simulink model "ebbers_moll_3"  (Simulink 7.4)
settings: Solver=ode23t  StartTime=0.0  StopTime=1e-6  MaxStep=1e-7  RelTol=1e-5
libraries: powerlib x71, simulink x1
settings Model: Creator=Dick Benson  LastModifiedBy=Dick
settings SolverCC: ZeroCrossControl=EnableAll
settings OptimizationCC: InlineInvariantSignals=on  InitFltsAndDblsToZero=on
settings DebuggingCC: AlgebraicLoopMsg=none  SaveWithParameterizedLinksMsg=none  SignalResolutionControl=TryResolveAllWithWarning  MultiTaskDSMMsg=warning  MultiTaskCondExecSysMsg=none  StrictBusMsg=None
settings RTWCC: IncludeERTFirstTime=on
settings GRTTargetCC: TargetFcnLib=ansi_tfl_tmw.mat

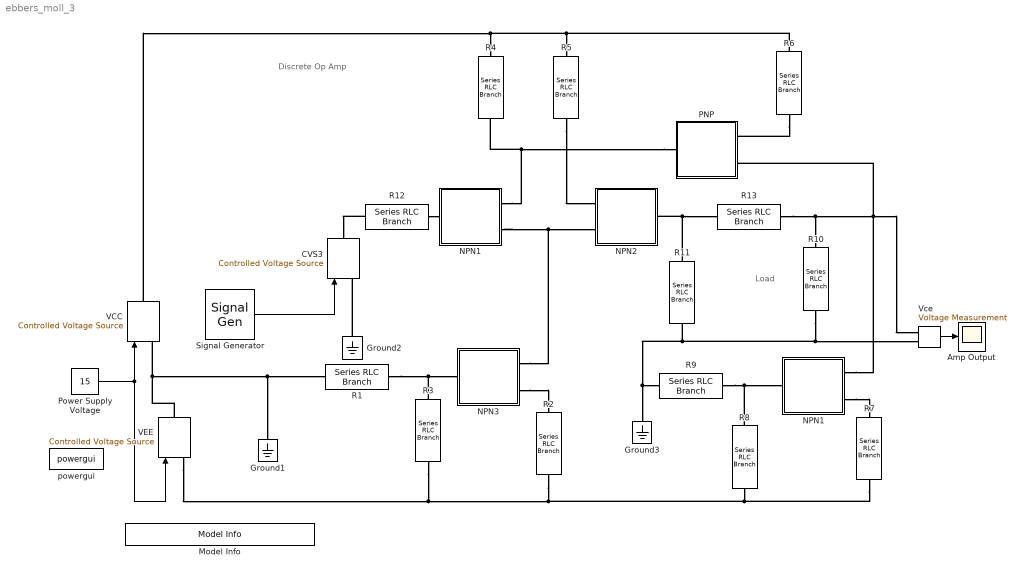
== system ebbers_moll_3 ==
  note: Discrete Op Amp
  note: Load
  " Power Supply Voltage" : Constant  Value=15  OutDataType=sfix(16)  OutScaling=2^0
  Amp Output : Scope
      settings: TimeRange=1e-006  YMin=-1.86228  YMax=1.74251  MaxDataPoints=50000
  CVS3 : powerlib/Electrical Sources/Controlled Voltage Source  DialogController=POWERSYS.PowerSysDialog  SystemSampleTime=-1  Initialize=on  Source_Type=AC  Amplitude=0  Phase=0  Frequency=0  Measurements=None
  Ground1 : powerlib/Elements/Ground  DialogController=POWERSYS.PowerSysDialog  PhysicalDomain=powersysdomain  SubClassName=unknown  LeftPortType=p1  RightPortType=p1  LConnTagsString=a
  Ground2 : powerlib/Elements/Ground  DialogController=POWERSYS.PowerSysDialog  PhysicalDomain=powersysdomain  SubClassName=unknown  LeftPortType=p1  RightPortType=p1  LConnTagsString=a
  Ground3 : powerlib/Elements/Ground  DialogController=POWERSYS.PowerSysDialog  PhysicalDomain=powersysdomain  SubClassName=unknown  LeftPortType=p1  RightPortType=p1  LConnTagsString=a
  Model Info : simulink/Model-Wide Utilities/Model Info  SystemSampleTime=-1  InitialBlockCM=None  BlockCM=None  Frame=on  DisplayStringWithTags=Copywrite 2005-2010 The MathWorks, Inc.  HorizontalTextAlignment=Center  LeftAlignmentValue=0.5  SourceBlockDiagram=ebbers_moll_3  TagMaxNumber=20
  NPN1 : Subsystem  mask{Beta=100, IEs=1e-10;, ICs=1e-10;, Ro=1e5, Cbc=5e-12, Cbe=50e-12, Rbb=100}
      mask init:
      | k = 1.38e-23;
      | q = 1.6e-19;
      | T = 290;
      | Vt = k*T/q;
  "NPN1 " : Subsystem  mask{Beta=40, IEs=1e-10;, ICs=1e-10;, Ro=1e5, Cbc=5e-12, Cbe=50e-12, Rbb=100}
      mask init:
      | k = 1.38e-23;
      | q = 1.6e-19;
      | T = 290;
      | Vt = k*T/q;
  NPN2 : Subsystem  mask{Beta=40, IEs=1e-10;, ICs=1e-10;, Ro=1e5, Cbc=5e-12, Cbe=50e-12, Rbb=100}
      mask init:
      | k = 1.38e-23;
      | q = 1.6e-19;
      | T = 290;
      | Vt = k*T/q;
  NPN3 : Subsystem  mask{Beta=100, IEs=1e-10;, ICs=1e-10;, Ro=1e5, Cbc=5e-12, Cbe=50e-12, Rbb=100}
      mask init:
      | k = 1.38e-23;
      | q = 1.6e-19;
      | T = 290;
      | Vt = k*T/q;
  PNP : Subsystem  mask{Beta=100, IEs=1e-8;, ICs=1e-8;, Ro=1e5, Cbc=5e-12, Cbe=50e-12, Rbb=100}
      mask init:
      | k = 1.38e-23;
      | q = 1.6e-19;
      | T = 290;
      | Vt = k*T/q;
  R{1,3,8..9} (4 alike) : powerlib/Elements/Series RLC Branch  DialogController=POWERSYS.PowerSysDialog  PhysicalDomain=powersysdomain  SubClassName=unknown  LeftPortType=p1  RightPortType=p1  LConnTagsString=__new0  RConnTagsString=__new0  BranchType=R  Resistance=1000  Inductance=1.0  SetiL0=off  InitialCurrent=0  Capacitance=1.0  Setx0=off  InitialVoltage=0  Measurements=None
  R10 : powerlib/Elements/Series RLC Branch  DialogController=POWERSYS.PowerSysDialog  PhysicalDomain=powersysdomain  SubClassName=unknown  LeftPortType=p1  RightPortType=p1  LConnTagsString=__new0  RConnTagsString=__new0  BranchType=R  Resistance=50  Inductance=1.0  SetiL0=off  InitialCurrent=0  Capacitance=1.0  Setx0=off  InitialVoltage=0  Measurements=None
  R11 : powerlib/Elements/Series RLC Branch  DialogController=POWERSYS.PowerSysDialog  PhysicalDomain=powersysdomain  SubClassName=unknown  LeftPortType=p1  RightPortType=p1  LConnTagsString=__new0  RConnTagsString=__new0  BranchType=R  Resistance=250  Inductance=1.0  SetiL0=off  InitialCurrent=0  Capacitance=1.0  Setx0=off  InitialVoltage=0  Measurements=None
  R12 : powerlib/Elements/Series RLC Branch  DialogController=POWERSYS.PowerSysDialog  PhysicalDomain=powersysdomain  SubClassName=unknown  LeftPortType=p1  RightPortType=p1  LConnTagsString=__new0  RConnTagsString=__new0  BranchType=R  Resistance=200  Inductance=1.0  SetiL0=off  InitialCurrent=0  Capacitance=1.0  Setx0=off  InitialVoltage=0  Measurements=None
  R13 : powerlib/Elements/Series RLC Branch  DialogController=POWERSYS.PowerSysDialog  PhysicalDomain=powersysdomain  SubClassName=unknown  LeftPortType=p1  RightPortType=p1  LConnTagsString=__new0  RConnTagsString=__new0  BranchType=R  Resistance=1200  Inductance=1.0  SetiL0=off  InitialCurrent=0  Capacitance=1.0  Setx0=off  InitialVoltage=0  Measurements=None
  R2 : powerlib/Elements/Series RLC Branch  DialogController=POWERSYS.PowerSysDialog  PhysicalDomain=powersysdomain  SubClassName=unknown  LeftPortType=p1  RightPortType=p1  LConnTagsString=__new0  RConnTagsString=__new0  BranchType=R  Resistance=330  Inductance=1.0  SetiL0=off  InitialCurrent=0  Capacitance=1.0  Setx0=off  InitialVoltage=0  Measurements=None
  R4 : powerlib/Elements/Series RLC Branch  DialogController=POWERSYS.PowerSysDialog  PhysicalDomain=powersysdomain  SubClassName=unknown  LeftPortType=p1  RightPortType=p1  LConnTagsString=__new0  RConnTagsString=__new0  BranchType=R  Resistance=200  Inductance=1.0  SetiL0=off  InitialCurrent=0  Capacitance=1.0  Setx0=off  InitialVoltage=0  Measurements=None
  R5 : powerlib/Elements/Series RLC Branch  DialogController=POWERSYS.PowerSysDialog  PhysicalDomain=powersysdomain  SubClassName=unknown  LeftPortType=p1  RightPortType=p1  LConnTagsString=__new0  RConnTagsString=__new0  BranchType=R  Resistance=200  Inductance=1.0  SetiL0=off  InitialCurrent=0  Capacitance=1.0  Setx0=off  InitialVoltage=0  Measurements=None
  R6 : powerlib/Elements/Series RLC Branch  DialogController=POWERSYS.PowerSysDialog  PhysicalDomain=powersysdomain  SubClassName=unknown  LeftPortType=p1  RightPortType=p1  LConnTagsString=__new0  RConnTagsString=__new0  BranchType=R  Resistance=10  Inductance=1.0  SetiL0=off  InitialCurrent=0  Capacitance=1.0  Setx0=off  InitialVoltage=0  Measurements=None
  R7 : powerlib/Elements/Series RLC Branch  DialogController=POWERSYS.PowerSysDialog  PhysicalDomain=powersysdomain  SubClassName=unknown  LeftPortType=p1  RightPortType=p1  LConnTagsString=__new0  RConnTagsString=__new0  BranchType=R  Resistance=50.35  Inductance=1.0  SetiL0=off  InitialCurrent=0  Capacitance=1.0  Setx0=off  InitialVoltage=0  Measurements=None
  Signal Generator : SignalGenerator  WaveForm=square  Amplitude=.2  Frequency=1e6
  VCC : powerlib/Electrical Sources/Controlled Voltage Source  DialogController=POWERSYS.PowerSysDialog  SystemSampleTime=-1  Initialize=on  Source_Type=DC  Amplitude=0  Phase=0  Frequency=0  Measurements=None
  VEE : powerlib/Electrical Sources/Controlled Voltage Source  DialogController=POWERSYS.PowerSysDialog  SystemSampleTime=-1  Initialize=on  Source_Type=DC  Amplitude=0  Phase=0  Frequency=0  Measurements=None
  "Vce " : powerlib/Measurements/Voltage Measurement  DialogController=POWERSYS.PowerSysDialog  SystemSampleTime=-1  PhasorSimulation=off  OutputType=Complex  PSBequivalent=0
  powergui : powerlib/powergui  SystemSampleTime=-1  SimulationMode=Continuous  SampleTime=0  frequency=60  SPID=off  DisableSnubberDevices=off  DisableRonSwitches=off  DisableVfSwitches=off  SwTol=0  Interpol=off  frequencyindice=0  echomessages=off  HookPort=off  DisplayEquations=off  FunctionMessages=off  EnableUseOfTLC=off  x0status=blocks  RestoreLinks=warning  Frange=[0:2:500]  Ylog=off  Xlog=on  ShowGrid=off  save=off  variable=ZData  ZoomFFT=on  StartTime=0.0  cycles=1  DisplayStyle=1  fundamental=60  FreqAxis=off  MaxFrequency=1000  frequencyindicesteady=1  RmsSteady=1  display=off  Ts=0  methode=off
  wires:
  "Vce "/1 -> Amp Output/1
  " Power Supply Voltage"/1 -> VCC/1, VEE/1
  Signal Generator/1 -> CVS3/1
  connections:
  VEE/LConn1 -- R7/RConn1 -- R8/RConn1 -- R2/RConn1 -- R3/RConn1
  NPN3/RConn2 -- R2/LConn1
  R3/LConn1 -- NPN3/LConn1 -- R1/RConn1
  "NPN1 "/RConn2 -- NPN2/RConn2 -- NPN3/RConn1
  PNP/LConn1 -- "NPN1 "/RConn1 -- R4/RConn1
  R5/RConn1 -- NPN2/RConn1
  R6/LConn1 -- VCC/RConn1 -- R4/LConn1 -- R5/LConn1
  VEE/RConn1 -- VCC/LConn1 -- R1/LConn1 -- Ground1/LConn1
  Ground2/LConn1 -- CVS3/LConn1
  R6/RConn1 -- PNP/RConn1
  R11/RConn1 -- R10/RConn1 -- "Vce "/LConn2 -- Ground3/LConn1 -- R9/LConn1
  NPN1/RConn2 -- R7/LConn1
  R8/LConn1 -- NPN1/LConn1 -- R9/RConn1
  R11/LConn1 -- NPN2/LConn1 -- R13/LConn1
  R12/LConn1 -- "NPN1 "/LConn1
  R12/RConn1 -- CVS3/RConn1
  R10/LConn1 -- R13/RConn1 -- PNP/RConn2 -- NPN1/RConn1 -- "Vce "/LConn1

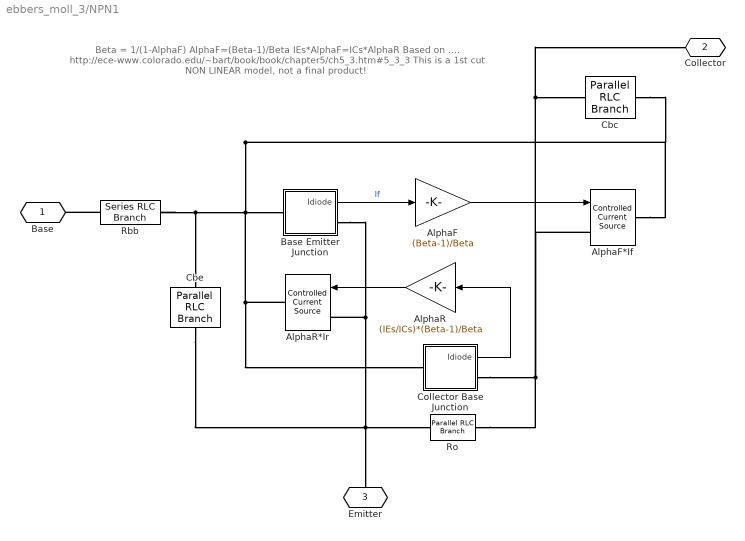
== system ebbers_moll_3/NPN1 ==
  note: Beta = 1/(1-AlphaF)
      | AlphaF=(Beta-1)/Beta
      | IEs*AlphaF=ICs*AlphaR
      |
      | Based on ....
      | http://ece-www.colorado.edu/~bart/book/book/chapter5/ch5_3.htm#5_3_3
      |
      | This is a 1st cut NON LINEAR model, not a final product!
  AlphaF : Gain  Gain=(Beta-1)/Beta  ParameterDataType=sfix(16)  ParameterScaling=2^0  OutDataType=sfix(16)  OutScaling=2^0
  AlphaF*If : powerlib/Electrical Sources/Controlled Current Source  Description=source block  DialogController=POWERSYS.PowerSysDialog  SystemSampleTime=-1  Initialize=off  Source_Type=AC  Amplitude=-0.025  Phase=0  Frequency=0  Measurements=None
      settings: AttributesFormatString=\n
  AlphaR : Gain  Gain=(IEs/ICs)*(Beta-1)/Beta  ParameterDataType=sfix(16)  ParameterScaling=2^0  OutDataType=sfix(16)  OutScaling=2^0
  AlphaR*Ir : powerlib/Electrical Sources/Controlled Current Source  Description=source block  DialogController=POWERSYS.PowerSysDialog  SystemSampleTime=-1  Initialize=off  Source_Type=AC  Amplitude=-0.025  Phase=0  Frequency=0  Measurements=None
      settings: AttributesFormatString=\n
  Base Emitter Junction : Subsystem  AncestorBlock=simcircuits_library_1/diode  mask{Is=IEs}
      mask prompts: Is "Saturation Current"
      mask Display: plot(-140,-140,150,140,2*[30,30,59,30,30,0]-75,(2*[71,50,72,92,71,71]-92),2*[59,59]-75,(2*[50,93]-92),[116,59]-16,(2*[71,71]-90));
  Cbc : powerlib/Elements/Parallel RLC Branch  DialogController=POWERSYS.PowerSysDialog  PhysicalDomain=powersysdomain  SubClassName=unknown  LeftPortType=p1  RightPortType=p1  LConnTagsString=a  RConnTagsString=__new0  BranchType=C  Resistance=1.0  Inductance=1.0  SetiL0=off  InitialCurrent=0  Capacitance=Cbc  Setx0=off  InitialVoltage=0  Measurements=None
  Cbe : powerlib/Elements/Parallel RLC Branch  DialogController=POWERSYS.PowerSysDialog  PhysicalDomain=powersysdomain  SubClassName=unknown  LeftPortType=p1  RightPortType=p1  LConnTagsString=a  RConnTagsString=__new0  BranchType=C  Resistance=1.0  Inductance=1.0  SetiL0=off  InitialCurrent=0  Capacitance=Cbe  Setx0=off  InitialVoltage=0  Measurements=None
  Collector Base Junction : Subsystem  AncestorBlock=simcircuits_library_1/diode  mask{Is=ICs}
      mask prompts: Is "Saturation Current"
      mask Display: plot(-140,-140,150,140,2*[30,30,59,30,30,0]-75,(2*[71,50,72,92,71,71]-92),2*[59,59]-75,(2*[50,93]-92),[116,59]-16,(2*[71,71]-90));
  Rbb : powerlib/Elements/Series RLC Branch  DialogController=POWERSYS.PowerSysDialog  PhysicalDomain=powersysdomain  SubClassName=unknown  LeftPortType=p1  RightPortType=p1  LConnTagsString=__new0  RConnTagsString=__new0  BranchType=R  Resistance=Rbb  Inductance=1.0  SetiL0=off  InitialCurrent=0  Capacitance=1.0  Setx0=off  InitialVoltage=0  Measurements=None
  Ro : powerlib/Elements/Parallel RLC Branch  DialogController=POWERSYS.PowerSysDialog  PhysicalDomain=powersysdomain  SubClassName=unknown  LeftPortType=p1  RightPortType=p1  LConnTagsString=a  RConnTagsString=__new0  BranchType=R  Resistance=Ro  Inductance=1.0  SetiL0=off  InitialCurrent=0  Capacitance=1.0  Setx0=off  InitialVoltage=0  Measurements=None
  Base : PMIOPort  Port=1  Side=Left
  Collector : PMIOPort  Port=2  Side=Right
  Emitter : PMIOPort  Port=3  Side=Right
  wires:
  Base Emitter Junction/1(Idiode) -> AlphaF/1  "If"
  AlphaF/1 -> AlphaF*If/1
  Collector Base Junction/1(Idiode) -> AlphaR/1
  AlphaR/1 -> AlphaR*Ir/1
  connections:
  Rbb/RConn1 -- Cbe/LConn1 -- Base Emitter Junction/LConn1 -- AlphaF*If/RConn1 -- Cbc/RConn1 -- AlphaR*Ir/RConn1 -- Collector Base Junction/LConn1
  AlphaR*Ir/LConn1 -- Emitter/RConn1 -- Cbe/RConn1 -- Ro/LConn1 -- Base Emitter Junction/RConn1
  AlphaF*If/LConn1 -- Collector/RConn1 -- Cbc/LConn1 -- Collector Base Junction/RConn1 -- Ro/RConn1
  Rbb/LConn1 -- Base/RConn1

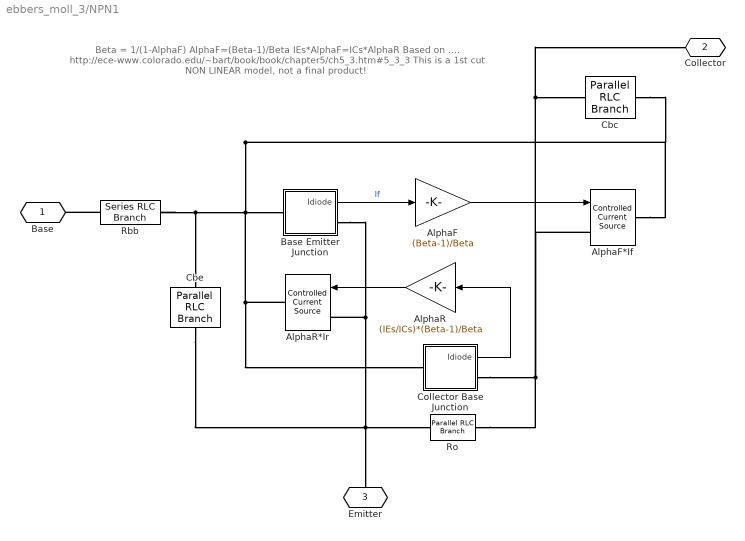
== system ebbers_moll_3/NPN1  ==
  note: Beta = 1/(1-AlphaF)
      | AlphaF=(Beta-1)/Beta
      | IEs*AlphaF=ICs*AlphaR
      |
      | Based on ....
      | http://ece-www.colorado.edu/~bart/book/book/chapter5/ch5_3.htm#5_3_3
      |
      | This is a 1st cut NON LINEAR model, not a final product!
  AlphaF : Gain  Gain=(Beta-1)/Beta  ParameterDataType=sfix(16)  ParameterScaling=2^0  OutDataType=sfix(16)  OutScaling=2^0
  AlphaF*If : powerlib/Electrical Sources/Controlled Current Source  Description=source block  DialogController=POWERSYS.PowerSysDialog  SystemSampleTime=-1  Initialize=off  Source_Type=AC  Amplitude=-0.025  Phase=0  Frequency=0  Measurements=None
      settings: AttributesFormatString=\n
  AlphaR : Gain  Gain=(IEs/ICs)*(Beta-1)/Beta  ParameterDataType=sfix(16)  ParameterScaling=2^0  OutDataType=sfix(16)  OutScaling=2^0
  AlphaR*Ir : powerlib/Electrical Sources/Controlled Current Source  Description=source block  DialogController=POWERSYS.PowerSysDialog  SystemSampleTime=-1  Initialize=off  Source_Type=AC  Amplitude=-0.025  Phase=0  Frequency=0  Measurements=None
      settings: AttributesFormatString=\n
  Base Emitter Junction : Subsystem  AncestorBlock=simcircuits_library_1/diode  mask{Is=IEs}
      mask prompts: Is "Saturation Current"
      mask Display: plot(-140,-140,150,140,2*[30,30,59,30,30,0]-75,(2*[71,50,72,92,71,71]-92),2*[59,59]-75,(2*[50,93]-92),[116,59]-16,(2*[71,71]-90));
  Cbc : powerlib/Elements/Parallel RLC Branch  DialogController=POWERSYS.PowerSysDialog  PhysicalDomain=powersysdomain  SubClassName=unknown  LeftPortType=p1  RightPortType=p1  LConnTagsString=a  RConnTagsString=__new0  BranchType=C  Resistance=1.0  Inductance=1.0  SetiL0=off  InitialCurrent=0  Capacitance=Cbc  Setx0=off  InitialVoltage=0  Measurements=None
  Cbe : powerlib/Elements/Parallel RLC Branch  DialogController=POWERSYS.PowerSysDialog  PhysicalDomain=powersysdomain  SubClassName=unknown  LeftPortType=p1  RightPortType=p1  LConnTagsString=a  RConnTagsString=__new0  BranchType=C  Resistance=1.0  Inductance=1.0  SetiL0=off  InitialCurrent=0  Capacitance=Cbe  Setx0=off  InitialVoltage=0  Measurements=None
  Collector Base Junction : Subsystem  AncestorBlock=simcircuits_library_1/diode  mask{Is=ICs}
      mask prompts: Is "Saturation Current"
      mask Display: plot(-140,-140,150,140,2*[30,30,59,30,30,0]-75,(2*[71,50,72,92,71,71]-92),2*[59,59]-75,(2*[50,93]-92),[116,59]-16,(2*[71,71]-90));
  Rbb : powerlib/Elements/Series RLC Branch  DialogController=POWERSYS.PowerSysDialog  PhysicalDomain=powersysdomain  SubClassName=unknown  LeftPortType=p1  RightPortType=p1  LConnTagsString=__new0  RConnTagsString=__new0  BranchType=R  Resistance=Rbb  Inductance=1.0  SetiL0=off  InitialCurrent=0  Capacitance=1.0  Setx0=off  InitialVoltage=0  Measurements=None
  Ro : powerlib/Elements/Parallel RLC Branch  DialogController=POWERSYS.PowerSysDialog  PhysicalDomain=powersysdomain  SubClassName=unknown  LeftPortType=p1  RightPortType=p1  LConnTagsString=a  RConnTagsString=__new0  BranchType=R  Resistance=Ro  Inductance=1.0  SetiL0=off  InitialCurrent=0  Capacitance=1.0  Setx0=off  InitialVoltage=0  Measurements=None
  Base : PMIOPort  Port=1  Side=Left
  Collector : PMIOPort  Port=2  Side=Right
  Emitter : PMIOPort  Port=3  Side=Right
  wires:
  Base Emitter Junction/1(Idiode) -> AlphaF/1  "If"
  AlphaF/1 -> AlphaF*If/1
  Collector Base Junction/1(Idiode) -> AlphaR/1
  AlphaR/1 -> AlphaR*Ir/1
  connections:
  Rbb/RConn1 -- Cbe/LConn1 -- Base Emitter Junction/LConn1 -- AlphaF*If/RConn1 -- Cbc/RConn1 -- AlphaR*Ir/RConn1 -- Collector Base Junction/LConn1
  AlphaR*Ir/LConn1 -- Emitter/RConn1 -- Cbe/RConn1 -- Ro/LConn1 -- Base Emitter Junction/RConn1
  AlphaF*If/LConn1 -- Collector/RConn1 -- Cbc/LConn1 -- Collector Base Junction/RConn1 -- Ro/RConn1
  Rbb/LConn1 -- Base/RConn1

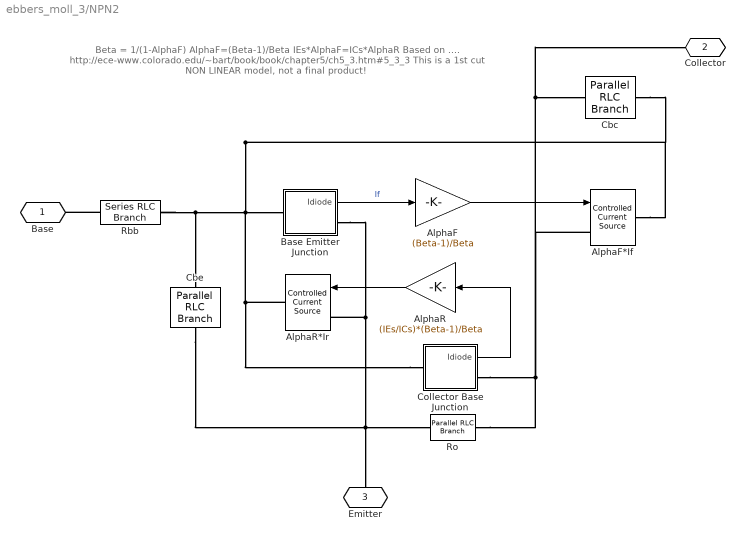
== system ebbers_moll_3/NPN2 ==
  note: Beta = 1/(1-AlphaF)
      | AlphaF=(Beta-1)/Beta
      | IEs*AlphaF=ICs*AlphaR
      |
      | Based on ....
      | http://ece-www.colorado.edu/~bart/book/book/chapter5/ch5_3.htm#5_3_3
      |
      | This is a 1st cut NON LINEAR model, not a final product!
  AlphaF : Gain  Gain=(Beta-1)/Beta  ParameterDataType=sfix(16)  ParameterScaling=2^0  OutDataType=sfix(16)  OutScaling=2^0
  AlphaF*If : powerlib/Electrical Sources/Controlled Current Source  Description=source block  DialogController=POWERSYS.PowerSysDialog  SystemSampleTime=-1  Initialize=off  Source_Type=AC  Amplitude=-0.025  Phase=0  Frequency=0  Measurements=None
      settings: AttributesFormatString=\n
  AlphaR : Gain  Gain=(IEs/ICs)*(Beta-1)/Beta  ParameterDataType=sfix(16)  ParameterScaling=2^0  OutDataType=sfix(16)  OutScaling=2^0
  AlphaR*Ir : powerlib/Electrical Sources/Controlled Current Source  Description=source block  DialogController=POWERSYS.PowerSysDialog  SystemSampleTime=-1  Initialize=off  Source_Type=AC  Amplitude=-0.025  Phase=0  Frequency=0  Measurements=None
      settings: AttributesFormatString=\n
  Base Emitter Junction : Subsystem  AncestorBlock=simcircuits_library_1/diode  mask{Is=IEs}
      mask prompts: Is "Saturation Current"
      mask Display: plot(-140,-140,150,140,2*[30,30,59,30,30,0]-75,(2*[71,50,72,92,71,71]-92),2*[59,59]-75,(2*[50,93]-92),[116,59]-16,(2*[71,71]-90));
  Cbc : powerlib/Elements/Parallel RLC Branch  DialogController=POWERSYS.PowerSysDialog  PhysicalDomain=powersysdomain  SubClassName=unknown  LeftPortType=p1  RightPortType=p1  LConnTagsString=a  RConnTagsString=__new0  BranchType=C  Resistance=1.0  Inductance=1.0  SetiL0=off  InitialCurrent=0  Capacitance=Cbc  Setx0=off  InitialVoltage=0  Measurements=None
  Cbe : powerlib/Elements/Parallel RLC Branch  DialogController=POWERSYS.PowerSysDialog  PhysicalDomain=powersysdomain  SubClassName=unknown  LeftPortType=p1  RightPortType=p1  LConnTagsString=a  RConnTagsString=__new0  BranchType=C  Resistance=1.0  Inductance=1.0  SetiL0=off  InitialCurrent=0  Capacitance=Cbe  Setx0=off  InitialVoltage=0  Measurements=None
  Collector Base Junction : Subsystem  AncestorBlock=simcircuits_library_1/diode  mask{Is=ICs}
      mask prompts: Is "Saturation Current"
      mask Display: plot(-140,-140,150,140,2*[30,30,59,30,30,0]-75,(2*[71,50,72,92,71,71]-92),2*[59,59]-75,(2*[50,93]-92),[116,59]-16,(2*[71,71]-90));
  Rbb : powerlib/Elements/Series RLC Branch  DialogController=POWERSYS.PowerSysDialog  PhysicalDomain=powersysdomain  SubClassName=unknown  LeftPortType=p1  RightPortType=p1  LConnTagsString=__new0  RConnTagsString=__new0  BranchType=R  Resistance=Rbb  Inductance=1.0  SetiL0=off  InitialCurrent=0  Capacitance=1.0  Setx0=off  InitialVoltage=0  Measurements=None
  Ro : powerlib/Elements/Parallel RLC Branch  DialogController=POWERSYS.PowerSysDialog  PhysicalDomain=powersysdomain  SubClassName=unknown  LeftPortType=p1  RightPortType=p1  LConnTagsString=a  RConnTagsString=__new0  BranchType=R  Resistance=Ro  Inductance=1.0  SetiL0=off  InitialCurrent=0  Capacitance=1.0  Setx0=off  InitialVoltage=0  Measurements=None
  Base : PMIOPort  Port=1  Side=Left
  Collector : PMIOPort  Port=2  Side=Right
  Emitter : PMIOPort  Port=3  Side=Right
  wires:
  AlphaR/1 -> AlphaR*Ir/1
  Collector Base Junction/1(Idiode) -> AlphaR/1
  AlphaF/1 -> AlphaF*If/1
  Base Emitter Junction/1(Idiode) -> AlphaF/1  "If"
  connections:
  Rbb/LConn1 -- Base/RConn1
  Ro/RConn1 -- Collector Base Junction/RConn1 -- Cbc/LConn1 -- Collector/RConn1 -- AlphaF*If/LConn1
  Base Emitter Junction/RConn1 -- Ro/LConn1 -- Cbe/RConn1 -- Emitter/RConn1 -- AlphaR*Ir/LConn1
  Collector Base Junction/LConn1 -- AlphaR*Ir/RConn1 -- Cbc/RConn1 -- AlphaF*If/RConn1 -- Base Emitter Junction/LConn1 -- Cbe/LConn1 -- Rbb/RConn1

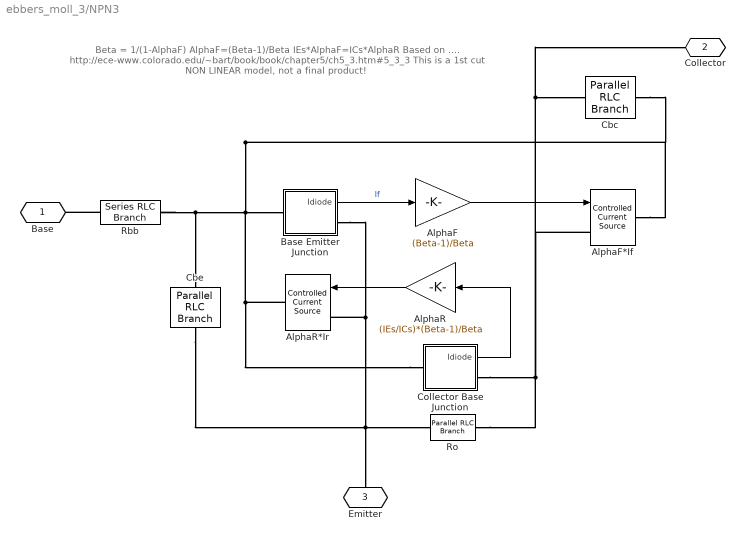
== system ebbers_moll_3/NPN3 ==
  note: Beta = 1/(1-AlphaF)
      | AlphaF=(Beta-1)/Beta
      | IEs*AlphaF=ICs*AlphaR
      |
      | Based on ....
      | http://ece-www.colorado.edu/~bart/book/book/chapter5/ch5_3.htm#5_3_3
      |
      | This is a 1st cut NON LINEAR model, not a final product!
  AlphaF : Gain  Gain=(Beta-1)/Beta  ParameterDataType=sfix(16)  ParameterScaling=2^0  OutDataType=sfix(16)  OutScaling=2^0
  AlphaF*If : powerlib/Electrical Sources/Controlled Current Source  Description=source block  DialogController=POWERSYS.PowerSysDialog  SystemSampleTime=-1  Initialize=off  Source_Type=AC  Amplitude=-0.025  Phase=0  Frequency=0  Measurements=None
      settings: AttributesFormatString=\n
  AlphaR : Gain  Gain=(IEs/ICs)*(Beta-1)/Beta  ParameterDataType=sfix(16)  ParameterScaling=2^0  OutDataType=sfix(16)  OutScaling=2^0
  AlphaR*Ir : powerlib/Electrical Sources/Controlled Current Source  Description=source block  DialogController=POWERSYS.PowerSysDialog  SystemSampleTime=-1  Initialize=off  Source_Type=AC  Amplitude=-0.025  Phase=0  Frequency=0  Measurements=None
      settings: AttributesFormatString=\n
  Base Emitter Junction : Subsystem  AncestorBlock=simcircuits_library_1/diode  mask{Is=IEs}
      mask prompts: Is "Saturation Current"
      mask Display: plot(-140,-140,150,140,2*[30,30,59,30,30,0]-75,(2*[71,50,72,92,71,71]-92),2*[59,59]-75,(2*[50,93]-92),[116,59]-16,(2*[71,71]-90));
  Cbc : powerlib/Elements/Parallel RLC Branch  DialogController=POWERSYS.PowerSysDialog  PhysicalDomain=powersysdomain  SubClassName=unknown  LeftPortType=p1  RightPortType=p1  LConnTagsString=a  RConnTagsString=__new0  BranchType=C  Resistance=1.0  Inductance=1.0  SetiL0=off  InitialCurrent=0  Capacitance=Cbc  Setx0=off  InitialVoltage=0  Measurements=None
  Cbe : powerlib/Elements/Parallel RLC Branch  DialogController=POWERSYS.PowerSysDialog  PhysicalDomain=powersysdomain  SubClassName=unknown  LeftPortType=p1  RightPortType=p1  LConnTagsString=a  RConnTagsString=__new0  BranchType=C  Resistance=1.0  Inductance=1.0  SetiL0=off  InitialCurrent=0  Capacitance=Cbe  Setx0=off  InitialVoltage=0  Measurements=None
  Collector Base Junction : Subsystem  AncestorBlock=simcircuits_library_1/diode  mask{Is=ICs}
      mask prompts: Is "Saturation Current"
      mask Display: plot(-140,-140,150,140,2*[30,30,59,30,30,0]-75,(2*[71,50,72,92,71,71]-92),2*[59,59]-75,(2*[50,93]-92),[116,59]-16,(2*[71,71]-90));
  Rbb : powerlib/Elements/Series RLC Branch  DialogController=POWERSYS.PowerSysDialog  PhysicalDomain=powersysdomain  SubClassName=unknown  LeftPortType=p1  RightPortType=p1  LConnTagsString=__new0  RConnTagsString=__new0  BranchType=R  Resistance=Rbb  Inductance=1.0  SetiL0=off  InitialCurrent=0  Capacitance=1.0  Setx0=off  InitialVoltage=0  Measurements=None
  Ro : powerlib/Elements/Parallel RLC Branch  DialogController=POWERSYS.PowerSysDialog  PhysicalDomain=powersysdomain  SubClassName=unknown  LeftPortType=p1  RightPortType=p1  LConnTagsString=a  RConnTagsString=__new0  BranchType=R  Resistance=Ro  Inductance=1.0  SetiL0=off  InitialCurrent=0  Capacitance=1.0  Setx0=off  InitialVoltage=0  Measurements=None
  Base : PMIOPort  Port=1  Side=Left
  Collector : PMIOPort  Port=2  Side=Right
  Emitter : PMIOPort  Port=3  Side=Right
  wires:
  AlphaR/1 -> AlphaR*Ir/1
  Collector Base Junction/1(Idiode) -> AlphaR/1
  AlphaF/1 -> AlphaF*If/1
  Base Emitter Junction/1(Idiode) -> AlphaF/1  "If"
  connections:
  Rbb/LConn1 -- Base/RConn1
  Ro/RConn1 -- Collector Base Junction/RConn1 -- Cbc/LConn1 -- Collector/RConn1 -- AlphaF*If/LConn1
  Base Emitter Junction/RConn1 -- Ro/LConn1 -- Cbe/RConn1 -- Emitter/RConn1 -- AlphaR*Ir/LConn1
  Collector Base Junction/LConn1 -- AlphaR*Ir/RConn1 -- Cbc/RConn1 -- AlphaF*If/RConn1 -- Base Emitter Junction/LConn1 -- Cbe/LConn1 -- Rbb/RConn1

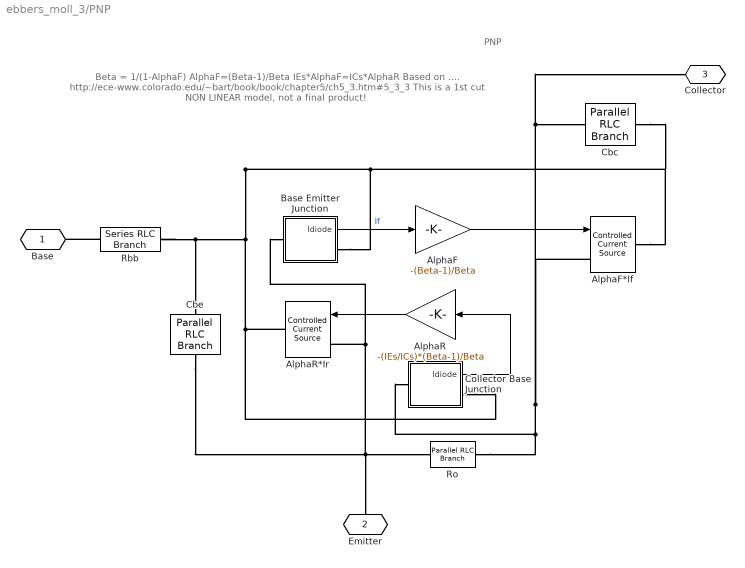
== system ebbers_moll_3/PNP ==
  note: Beta = 1/(1-AlphaF)
      | AlphaF=(Beta-1)/Beta
      | IEs*AlphaF=ICs*AlphaR
      |
      | Based on ....
      | http://ece-www.colorado.edu/~bart/book/book/chapter5/ch5_3.htm#5_3_3
      |
      | This is a 1st cut NON LINEAR model, not a final product!
  note: PNP
  AlphaF : Gain  Gain=-(Beta-1)/Beta  ParameterDataType=sfix(16)  ParameterScaling=2^0  OutDataType=sfix(16)  OutScaling=2^0
  AlphaF*If : powerlib/Electrical Sources/Controlled Current Source  Description=source block  DialogController=POWERSYS.PowerSysDialog  SystemSampleTime=-1  Initialize=off  Source_Type=AC  Amplitude=-0.025  Phase=0  Frequency=0  Measurements=None
      settings: AttributesFormatString=\n
  AlphaR : Gain  Gain=-(IEs/ICs)*(Beta-1)/Beta  ParameterDataType=sfix(16)  ParameterScaling=2^0  OutDataType=sfix(16)  OutScaling=2^0
  AlphaR*Ir : powerlib/Electrical Sources/Controlled Current Source  Description=source block  DialogController=POWERSYS.PowerSysDialog  SystemSampleTime=-1  Initialize=off  Source_Type=AC  Amplitude=-0.025  Phase=0  Frequency=0  Measurements=None
      settings: AttributesFormatString=\n
  Base Emitter Junction : Subsystem  AncestorBlock=simcircuits_library_1/diode  mask{Is=IEs}
      mask prompts: Is "Saturation Current"
      mask Display: plot(-140,-140,150,140,2*[30,30,59,30,30,0]-75,(2*[71,50,72,92,71,71]-92),2*[59,59]-75,(2*[50,93]-92),[116,59]-16,(2*[71,71]-90));
  Cbc : powerlib/Elements/Parallel RLC Branch  DialogController=POWERSYS.PowerSysDialog  PhysicalDomain=powersysdomain  SubClassName=unknown  LeftPortType=p1  RightPortType=p1  LConnTagsString=a  RConnTagsString=__new0  BranchType=C  Resistance=1.0  Inductance=1.0  SetiL0=off  InitialCurrent=0  Capacitance=Cbc  Setx0=off  InitialVoltage=0  Measurements=None
  Cbe : powerlib/Elements/Parallel RLC Branch  DialogController=POWERSYS.PowerSysDialog  PhysicalDomain=powersysdomain  SubClassName=unknown  LeftPortType=p1  RightPortType=p1  LConnTagsString=a  RConnTagsString=__new0  BranchType=C  Resistance=1.0  Inductance=1.0  SetiL0=off  InitialCurrent=0  Capacitance=Cbe  Setx0=off  InitialVoltage=0  Measurements=None
  Collector Base Junction : Subsystem  AncestorBlock=simcircuits_library_1/diode  mask{Is=ICs}
      mask prompts: Is "Saturation Current"
      mask Display: plot(-140,-140,150,140,2*[30,30,59,30,30,0]-75,(2*[71,50,72,92,71,71]-92),2*[59,59]-75,(2*[50,93]-92),[116,59]-16,(2*[71,71]-90));
  Rbb : powerlib/Elements/Series RLC Branch  DialogController=POWERSYS.PowerSysDialog  PhysicalDomain=powersysdomain  SubClassName=unknown  LeftPortType=p1  RightPortType=p1  LConnTagsString=__new0  RConnTagsString=__new0  BranchType=R  Resistance=Rbb  Inductance=1.0  SetiL0=off  InitialCurrent=0  Capacitance=1.0  Setx0=off  InitialVoltage=0  Measurements=None
  Ro : powerlib/Elements/Parallel RLC Branch  DialogController=POWERSYS.PowerSysDialog  PhysicalDomain=powersysdomain  SubClassName=unknown  LeftPortType=p1  RightPortType=p1  LConnTagsString=a  RConnTagsString=__new0  BranchType=R  Resistance=Ro  Inductance=1.0  SetiL0=off  InitialCurrent=0  Capacitance=1.0  Setx0=off  InitialVoltage=0  Measurements=None
  Base : PMIOPort  Port=1  Side=Left
  Emitter : PMIOPort  Port=2  Side=Right
  Collector : PMIOPort  Port=3  Side=Right
  wires:
  Base Emitter Junction/1(Idiode) -> AlphaF/1  "If"
  AlphaF/1 -> AlphaF*If/1
  Collector Base Junction/1(Idiode) -> AlphaR/1
  AlphaR/1 -> AlphaR*Ir/1
  connections:
  Collector Base Junction/RConn1 -- AlphaR*Ir/RConn1 -- Rbb/RConn1 -- Cbe/LConn1 -- AlphaF*If/RConn1 -- Cbc/RConn1 -- Base Emitter Junction/RConn1
  Emitter/RConn1 -- Cbe/RConn1 -- Ro/LConn1 -- AlphaR*Ir/LConn1 -- Base Emitter Junction/LConn1
  Ro/RConn1 -- AlphaF*If/LConn1 -- Collector/RConn1 -- Cbc/LConn1 -- Collector Base Junction/LConn1
  Rbb/LConn1 -- Base/RConn1

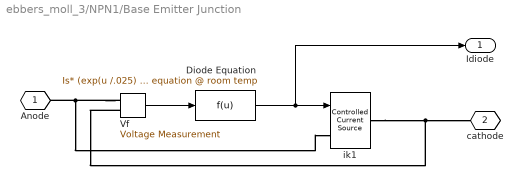
== system ebbers_moll_3/NPN1/Base Emitter Junction ==
  Diode Equation : Fcn  Expr="Is* (exp(u /.025)  -1  );  % ideal diode equation @ room temp"
  "Vf " : powerlib/Measurements/Voltage Measurement  Tag=PoWeRsYsTeMmEaSuReMeNt  DialogController=POWERSYS.PowerSysDialog  SystemSampleTime=-1  PhasorSimulation=off  OutputType=Magnitude  PSBequivalent=0
  ik1 : powerlib/Electrical Sources/Controlled Current Source  Description=source block  DialogController=POWERSYS.PowerSysDialog  SystemSampleTime=-1  Initialize=on  Source_Type=AC  Amplitude=0  Phase=0  Frequency=0  Measurements=None
      settings: AttributesFormatString=\n
  Anode : PMIOPort  Tag=PMCPort  Port=1  Side=Left
  "cathode " : PMIOPort  Tag=PMCPort  Port=2  Side=Right
  Idiode : Outport  OutDataType=sfix(16)  OutScaling=2^0
  wires:
  "Vf "/1 -> Diode Equation/1
  Diode Equation/1 -> ik1/1, Idiode/1
  connections:
  "Vf "/LConn1 -- Anode/RConn1 -- ik1/LConn1
  "Vf "/LConn2 -- "cathode "/RConn1 -- ik1/RConn1

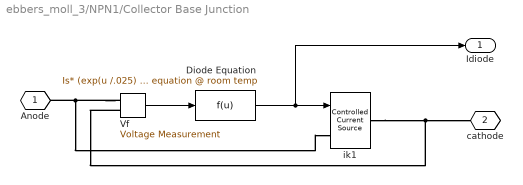
== system ebbers_moll_3/NPN1/Collector Base Junction ==
  Diode Equation : Fcn  Expr="Is* (exp(u /.025)  -1  );  % ideal diode equation @ room temp"
  "Vf " : powerlib/Measurements/Voltage Measurement  Tag=PoWeRsYsTeMmEaSuReMeNt  DialogController=POWERSYS.PowerSysDialog  SystemSampleTime=-1  PhasorSimulation=off  OutputType=Magnitude  PSBequivalent=0
  ik1 : powerlib/Electrical Sources/Controlled Current Source  Description=source block  DialogController=POWERSYS.PowerSysDialog  SystemSampleTime=-1  Initialize=on  Source_Type=AC  Amplitude=0  Phase=0  Frequency=0  Measurements=None
      settings: AttributesFormatString=\n
  Anode : PMIOPort  Tag=PMCPort  Port=1  Side=Left
  "cathode " : PMIOPort  Tag=PMCPort  Port=2  Side=Right
  Idiode : Outport  OutDataType=sfix(16)  OutScaling=2^0
  wires:
  Diode Equation/1 -> Idiode/1, ik1/1
  "Vf "/1 -> Diode Equation/1
  connections:
  ik1/RConn1 -- "cathode "/RConn1 -- "Vf "/LConn2
  ik1/LConn1 -- Anode/RConn1 -- "Vf "/LConn1

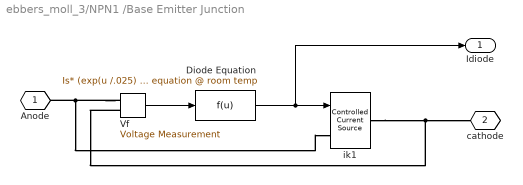
== system ebbers_moll_3/NPN1 /Base Emitter Junction ==
  Diode Equation : Fcn  Expr="Is* (exp(u /.025)  -1  );  % ideal diode equation @ room temp"
  "Vf " : powerlib/Measurements/Voltage Measurement  Tag=PoWeRsYsTeMmEaSuReMeNt  DialogController=POWERSYS.PowerSysDialog  SystemSampleTime=-1  PhasorSimulation=off  OutputType=Magnitude  PSBequivalent=0
  ik1 : powerlib/Electrical Sources/Controlled Current Source  Description=source block  DialogController=POWERSYS.PowerSysDialog  SystemSampleTime=-1  Initialize=on  Source_Type=AC  Amplitude=0  Phase=0  Frequency=0  Measurements=None
      settings: AttributesFormatString=\n
  Anode : PMIOPort  Tag=PMCPort  Port=1  Side=Left
  "cathode " : PMIOPort  Tag=PMCPort  Port=2  Side=Right
  Idiode : Outport  OutDataType=sfix(16)  OutScaling=2^0
  wires:
  "Vf "/1 -> Diode Equation/1
  Diode Equation/1 -> ik1/1, Idiode/1
  connections:
  "Vf "/LConn1 -- Anode/RConn1 -- ik1/LConn1
  "Vf "/LConn2 -- "cathode "/RConn1 -- ik1/RConn1

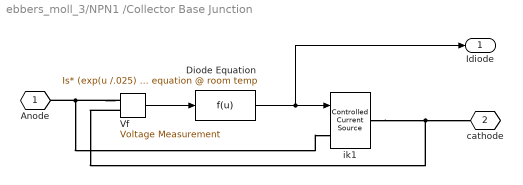
== system ebbers_moll_3/NPN1 /Collector Base Junction ==
  Diode Equation : Fcn  Expr="Is* (exp(u /.025)  -1  );  % ideal diode equation @ room temp"
  "Vf " : powerlib/Measurements/Voltage Measurement  Tag=PoWeRsYsTeMmEaSuReMeNt  DialogController=POWERSYS.PowerSysDialog  SystemSampleTime=-1  PhasorSimulation=off  OutputType=Magnitude  PSBequivalent=0
  ik1 : powerlib/Electrical Sources/Controlled Current Source  Description=source block  DialogController=POWERSYS.PowerSysDialog  SystemSampleTime=-1  Initialize=on  Source_Type=AC  Amplitude=0  Phase=0  Frequency=0  Measurements=None
      settings: AttributesFormatString=\n
  Anode : PMIOPort  Tag=PMCPort  Port=1  Side=Left
  "cathode " : PMIOPort  Tag=PMCPort  Port=2  Side=Right
  Idiode : Outport  OutDataType=sfix(16)  OutScaling=2^0
  wires:
  Diode Equation/1 -> Idiode/1, ik1/1
  "Vf "/1 -> Diode Equation/1
  connections:
  ik1/RConn1 -- "cathode "/RConn1 -- "Vf "/LConn2
  ik1/LConn1 -- Anode/RConn1 -- "Vf "/LConn1

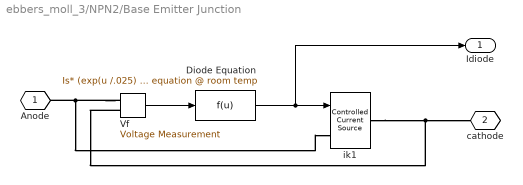
== system ebbers_moll_3/NPN2/Base Emitter Junction ==
  Diode Equation : Fcn  Expr="Is* (exp(u /.025)  -1  );  % ideal diode equation @ room temp"
  "Vf " : powerlib/Measurements/Voltage Measurement  Tag=PoWeRsYsTeMmEaSuReMeNt  DialogController=POWERSYS.PowerSysDialog  SystemSampleTime=-1  PhasorSimulation=off  OutputType=Magnitude  PSBequivalent=0
  ik1 : powerlib/Electrical Sources/Controlled Current Source  Description=source block  DialogController=POWERSYS.PowerSysDialog  SystemSampleTime=-1  Initialize=on  Source_Type=AC  Amplitude=0  Phase=0  Frequency=0  Measurements=None
      settings: AttributesFormatString=\n
  Anode : PMIOPort  Tag=PMCPort  Port=1  Side=Left
  "cathode " : PMIOPort  Tag=PMCPort  Port=2  Side=Right
  Idiode : Outport  OutDataType=sfix(16)  OutScaling=2^0
  wires:
  Diode Equation/1 -> Idiode/1, ik1/1
  "Vf "/1 -> Diode Equation/1
  connections:
  ik1/RConn1 -- "cathode "/RConn1 -- "Vf "/LConn2
  ik1/LConn1 -- Anode/RConn1 -- "Vf "/LConn1

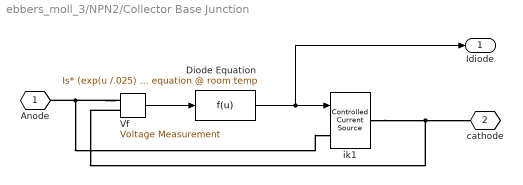
== system ebbers_moll_3/NPN2/Collector Base Junction ==
  Diode Equation : Fcn  Expr="Is* (exp(u /.025)  -1  );  % ideal diode equation @ room temp"
  "Vf " : powerlib/Measurements/Voltage Measurement  Tag=PoWeRsYsTeMmEaSuReMeNt  DialogController=POWERSYS.PowerSysDialog  SystemSampleTime=-1  PhasorSimulation=off  OutputType=Magnitude  PSBequivalent=0
  ik1 : powerlib/Electrical Sources/Controlled Current Source  Description=source block  DialogController=POWERSYS.PowerSysDialog  SystemSampleTime=-1  Initialize=on  Source_Type=AC  Amplitude=0  Phase=0  Frequency=0  Measurements=None
      settings: AttributesFormatString=\n
  Anode : PMIOPort  Tag=PMCPort  Port=1  Side=Left
  "cathode " : PMIOPort  Tag=PMCPort  Port=2  Side=Right
  Idiode : Outport  OutDataType=sfix(16)  OutScaling=2^0
  wires:
  "Vf "/1 -> Diode Equation/1
  Diode Equation/1 -> ik1/1, Idiode/1
  connections:
  "Vf "/LConn1 -- Anode/RConn1 -- ik1/LConn1
  "Vf "/LConn2 -- "cathode "/RConn1 -- ik1/RConn1

== system ebbers_moll_3/NPN3/Base Emitter Junction ==
  Diode Equation : Fcn  Expr="Is* (exp(u /.025)  -1  );  % ideal diode equation @ room temp"
  "Vf " : powerlib/Measurements/Voltage Measurement  Tag=PoWeRsYsTeMmEaSuReMeNt  DialogController=POWERSYS.PowerSysDialog  SystemSampleTime=-1  PhasorSimulation=off  OutputType=Magnitude  PSBequivalent=0
  ik1 : powerlib/Electrical Sources/Controlled Current Source  Description=source block  DialogController=POWERSYS.PowerSysDialog  SystemSampleTime=-1  Initialize=on  Source_Type=AC  Amplitude=0  Phase=0  Frequency=0  Measurements=None
      settings: AttributesFormatString=\n
  Anode : PMIOPort  Tag=PMCPort  Port=1  Side=Left
  "cathode " : PMIOPort  Tag=PMCPort  Port=2  Side=Right
  Idiode : Outport  OutDataType=sfix(16)  OutScaling=2^0
  wires:
  Diode Equation/1 -> Idiode/1, ik1/1
  "Vf "/1 -> Diode Equation/1
  connections:
  ik1/RConn1 -- "cathode "/RConn1 -- "Vf "/LConn2
  ik1/LConn1 -- Anode/RConn1 -- "Vf "/LConn1

== system ebbers_moll_3/NPN3/Collector Base Junction ==
  Diode Equation : Fcn  Expr="Is* (exp(u /.025)  -1  );  % ideal diode equation @ room temp"
  "Vf " : powerlib/Measurements/Voltage Measurement  Tag=PoWeRsYsTeMmEaSuReMeNt  DialogController=POWERSYS.PowerSysDialog  SystemSampleTime=-1  PhasorSimulation=off  OutputType=Magnitude  PSBequivalent=0
  ik1 : powerlib/Electrical Sources/Controlled Current Source  Description=source block  DialogController=POWERSYS.PowerSysDialog  SystemSampleTime=-1  Initialize=on  Source_Type=AC  Amplitude=0  Phase=0  Frequency=0  Measurements=None
      settings: AttributesFormatString=\n
  Anode : PMIOPort  Tag=PMCPort  Port=1  Side=Left
  "cathode " : PMIOPort  Tag=PMCPort  Port=2  Side=Right
  Idiode : Outport  OutDataType=sfix(16)  OutScaling=2^0
  wires:
  "Vf "/1 -> Diode Equation/1
  Diode Equation/1 -> ik1/1, Idiode/1
  connections:
  "Vf "/LConn1 -- Anode/RConn1 -- ik1/LConn1
  "Vf "/LConn2 -- "cathode "/RConn1 -- ik1/RConn1

== system ebbers_moll_3/PNP/Base Emitter Junction ==
  Diode Equation : Fcn  Expr="Is* (exp(u /.025)  -1  );  % ideal diode equation @ room temp"
  "Vf " : powerlib/Measurements/Voltage Measurement  Tag=PoWeRsYsTeMmEaSuReMeNt  DialogController=POWERSYS.PowerSysDialog  SystemSampleTime=-1  PhasorSimulation=off  OutputType=Magnitude  PSBequivalent=0
  ik1 : powerlib/Electrical Sources/Controlled Current Source  Description=source block  DialogController=POWERSYS.PowerSysDialog  SystemSampleTime=-1  Initialize=on  Source_Type=AC  Amplitude=0  Phase=0  Frequency=0  Measurements=None
      settings: AttributesFormatString=\n
  Anode : PMIOPort  Tag=PMCPort  Port=1  Side=Left
  "cathode " : PMIOPort  Tag=PMCPort  Port=2  Side=Right
  Idiode : Outport  OutDataType=sfix(16)  OutScaling=2^0
  wires:
  "Vf "/1 -> Diode Equation/1
  Diode Equation/1 -> ik1/1, Idiode/1
  connections:
  "Vf "/LConn1 -- Anode/RConn1 -- ik1/LConn1
  "Vf "/LConn2 -- "cathode "/RConn1 -- ik1/RConn1

== system ebbers_moll_3/PNP/Collector Base Junction ==
  Diode Equation : Fcn  Expr="Is* (exp(u /.025)  -1  );  % ideal diode equation @ room temp"
  "Vf " : powerlib/Measurements/Voltage Measurement  Tag=PoWeRsYsTeMmEaSuReMeNt  DialogController=POWERSYS.PowerSysDialog  SystemSampleTime=-1  PhasorSimulation=off  OutputType=Magnitude  PSBequivalent=0
  ik1 : powerlib/Electrical Sources/Controlled Current Source  Description=source block  DialogController=POWERSYS.PowerSysDialog  SystemSampleTime=-1  Initialize=on  Source_Type=AC  Amplitude=0  Phase=0  Frequency=0  Measurements=None
      settings: AttributesFormatString=\n
  Anode : PMIOPort  Tag=PMCPort  Port=1  Side=Left
  "cathode " : PMIOPort  Tag=PMCPort  Port=2  Side=Right
  Idiode : Outport  OutDataType=sfix(16)  OutScaling=2^0
  wires:
  Diode Equation/1 -> Idiode/1, ik1/1
  "Vf "/1 -> Diode Equation/1
  connections:
  ik1/RConn1 -- "cathode "/RConn1 -- "Vf "/LConn2
  ik1/LConn1 -- Anode/RConn1 -- "Vf "/LConn1
